simulink model "One_Pedal"  (R2024a)
settings: Solver=VariableStepAuto  StartTime=0.0  StopTime=10.0  RelTol=1e-3
undefined symbols (not defined in the file): Ion, Lithium
libraries: simulink x2, spsBatteryLib x1, spsControlledCurrentSourceLib x1, spsVoltageMeasurementLib x1, sps_lib x1
settings Model: Creator=ezeki  LastModifiedBy=ezeki

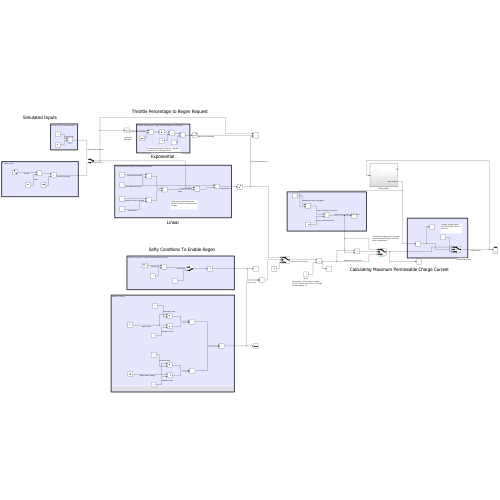
[thumbnail: Simulink's stored preview of the top-level diagram]
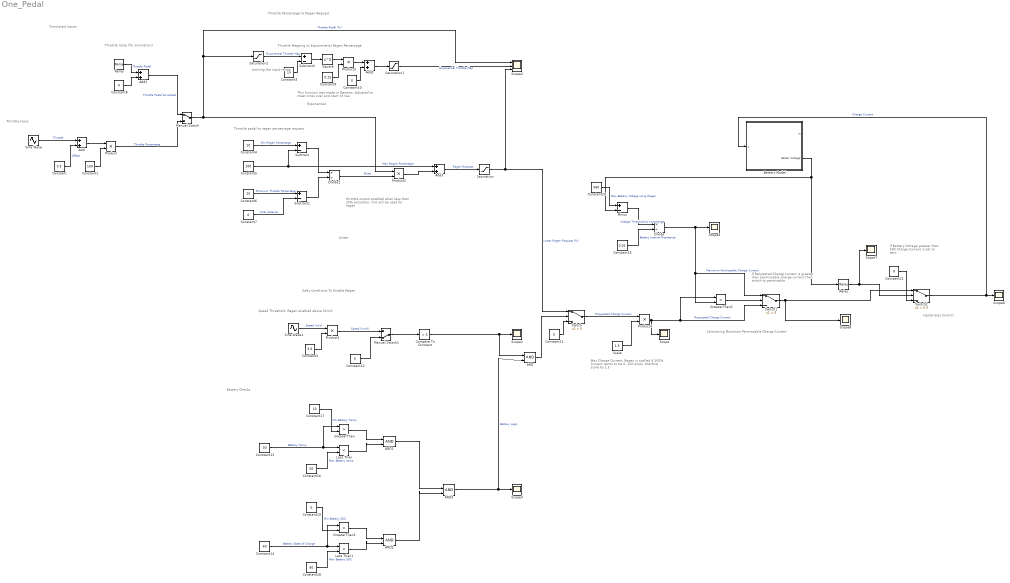
== system One_Pedal ==
  note: Linear
  note: Calculating Maximum Permissable Charge Current
  note: Throttle Percentage to Regen Request
  note: Simulated Inputs
  note: Safty Condtions To Enable Regen
  note: Max Charge Current, Regen is scalled 0-100%. Current wants to be 0 -150 amps, therfore scale by 1.5
  note: Battery Checks
  note: This function was made in Desmos. Adjusted to meet cross over and start of rise
  note: Limiting the input range
  note: Throttle Mapping to Exponenetial Regen Percentage
  note: Throttle ramp (for simulation)
  note: Throttle pedal to regen percentage request
  note: throttle output enabled when less then 20% actuation, this will be used for regen
  note: Speed Threshold, Regen enabled above 5km/h
  note: Throttle Input
  note: Hysterisies Control
  note: If Requested Charge current is greater then permissable charge current then switch to permisable
  note: If Battery Voltage greater then 590 Charge Current is set to zero
  note: Exponential
  AND{,1..3} (4 alike) : Logic  IconShape=distinctive  AllPortsSameDT=off  OutDataTypeStr=boolean
  Add{,1..3} (4 alike) : Sum
  Battery Model : Subsystem
  Compare To Constant : simulink/Logic and Bit Operations/Compare To Constant  relop=>  const=5  OutDataTypeStr=boolean
  Constant : Constant  Value=0.5
  Constant1 : Constant  Value=100
  Constant{7..8,10..11,21} (5 alike) : Constant  Value=0
  Constant12 : Constant  Value=6
  Constant13 : Constant  Value=30
  Constant14 : Constant  Value=60
  Constant15 : Constant  Value=0.01
  Constant16 : Constant  Value=50
  Constant17 : Constant  Value=10
  Constant18 : Constant  Value=90
  Constant19 : Constant  Value=5
  Constant2 : Constant  Value=3.6
  Constant20 : Constant  Value=580
  Constant3 : Constant  Value=20
  Constant4 : Constant  Value=10
  Constant5 : Constant  Value=100
  Constant6 : Constant  Value=20
  Constant9 : Constant  Value=0.25
  Divide : Product  Inputs=*/
  Divide1 : Product  Inputs=*/
  GreaterThan : RelationalOperator  Operator=>  OutDataTypeStr=boolean  RndMeth=Simplest  InputSameDT=off
  GreaterThan1 : RelationalOperator  Operator=>  OutDataTypeStr=boolean  RndMeth=Simplest  InputSameDT=off
  GreaterThan2 : RelationalOperator  Operator=>  OutDataTypeStr=boolean  RndMeth=Simplest  InputSameDT=off
  Less Than : RelationalOperator  Operator=<  OutDataTypeStr=boolean  RndMeth=Simplest  InputSameDT=off
  Less Than1 : RelationalOperator  Operator=<  OutDataTypeStr=boolean  RndMeth=Simplest  InputSameDT=off
  Manual Switch : ManualSwitch
  Manual Switch1 : ManualSwitch  CurrentSetting=0
  Minus : Sum  Inputs=+-
  Product{,1..4} (5 alike) : Product
  Ramp : simulink/Sources/Ramp  slope=-10  start=0  InitialOutput=100
  Relay : Relay  OnSwitchValue=590  OffSwitchValue=585  OnOutputValue=0  OffOutputValue=1
  Saturation : Saturate  UpperLimit=100  LowerLimit=0
  Saturation1 : Saturate  UpperLimit=100  LowerLimit=0
  Saturation2 : Saturate  UpperLimit=20  LowerLimit=0
  Scale : Constant  Value=1.5
  Scope{,1,3,6..9} (7 alike) : Scope
  Scope2 : Scope  NumInputPorts=3
  Sine Wave : Sin  Amplitude=0.5  SampleTime=0
  Sine Wave1 : Sin  SampleTime=0
  Square : Math  Operator=square
  Subtract : Sum  Inputs=+-
  Subtract1 : Sum  Inputs=+-
  Subtract2 : Sum  Inputs=+-
  Switch : Switch  Criteria=u2 > Threshold  SaturateOnIntegerOverflow=off  InputSameDT=off
  Switch1 : Switch  Criteria=u2 > Threshold  SaturateOnIntegerOverflow=off  InputSameDT=off
  Switch2 : Switch  Criteria=u2 > Threshold  Threshold=0.5  SaturateOnIntegerOverflow=off  InputSameDT=off
  wires:
  Sine Wave/1 -> Add/1  "Throttle"
  Constant/1 -> Add/2  "Offset"
  Constant1/1 -> Product/2
  Add/1 -> Product/1
  Product/1 -> Manual Switch/2  "Throttle Percentage"
  Sine Wave1/1 -> Product1/1  "Speed (m/s)"
  Constant2/1 -> Product1/2
  Product1/1 -> Manual Switch1/1  "Speed (km/h)"
  Compare To Constant/1 -> AND/1, Scope1/1
  Constant7/1 -> Subtract1/2  "Intial distance"
  Constant4/1 -> Subtract/1  "Min Regen Percentage"
  Constant6/1 -> Subtract1/1  "Minimum Throttle Percentage"
  Subtract/1 -> Divide1/1
  Constant5/1 -> Subtract/2, Add3/1  "Max Regen Percentage"
  Divide1/1 -> Product2/2  "Slope"
  Product2/1 -> Add3/2
  Subtract1/1 -> Divide1/2
  Add3/1 -> Saturation/1  "Regen Request"
  Manual Switch/1 -> Scope2/1, Saturation2/1, Product2/1  "Throttle Pedal (%)"
  Ramp/1 -> Add1/1  "Throttle Pedal"
  Constant8/1 -> Add1/2
  Add1/1 -> Manual Switch/1  "Throttle Pedal Simulated"
  Saturation/1 -> Switch/1, Scope2/3  "Linear Regen Request (%)"
  Subtract2/1 -> Square/1
  Constant3/1 -> Subtract2/2
  Add2/1 -> Saturation1/1
  Square/1 -> Product3/1
  Constant9/1 -> Product3/2
  Product3/1 -> Add2/1
  Constant10/1 -> Add2/2
  Saturation2/1 -> Subtract2/1  "Exponential Throttle Map"
  Constant11/1 -> Switch/3
  Manual Switch1/1 -> Compare To Constant/1
  Constant12/1 -> Manual Switch1/2
  AND/1 -> Switch/2
  Constant13/1 -> GreaterThan/1, Less Than/1  "Battery Temp"
  Constant14/1 -> GreaterThan1/1, Less Than1/1  "Battery State of Charge"
  AND3/1 -> Scope3/1, AND/2  "Battery Logic"
  Constant16/1 -> Less Than/2  "Max Battery temp"
  Constant17/1 -> GreaterThan/2  "Min Battery Temp"
  GreaterThan/1 -> AND1/1
  Less Than/1 -> AND1/2
  Constant19/1 -> GreaterThan1/2  "Min Battery SOC"
  GreaterThan1/1 -> AND2/1
  Constant18/1 -> Less Than1/2  "Max Battery SOC"
  Less Than1/1 -> AND2/2
  AND1/1 -> AND3/1
  AND2/1 -> AND3/2
  Switch2/1 -> Battery Model/1(s), Scope6/1  "Charge Current"
  Product4/1 -> Switch1/3, GreaterThan2/1, Scope/1  "Requested Charge Current"
  Divide/1 -> GreaterThan2/2, Switch1/1, Scope9/1  "Maximum Permissable Charge Current"
  Constant15/1 -> Divide/2  "Battery Internal Resistance"
  Battery Model/2(Batter Voltage) -> Minus/2, Relay/1
  Relay/1 -> Switch2/2, Scope7/1
  Constant21/1 -> Switch2/3
  Switch1/1 -> Switch2/1, Scope8/1
  Minus/1 -> Divide/1  "Voltage Threshold to overcharge"
  GreaterThan2/1 -> Switch1/2
  Constant20/1 -> Minus/1  "Max Battery Voltage using Regen"
  Switch/1 -> Product4/1  "Requested Charge Current"
  Scale/1 -> Product4/2
  Saturation1/1 -> Scope2/2  "Exponential Throttle Map"

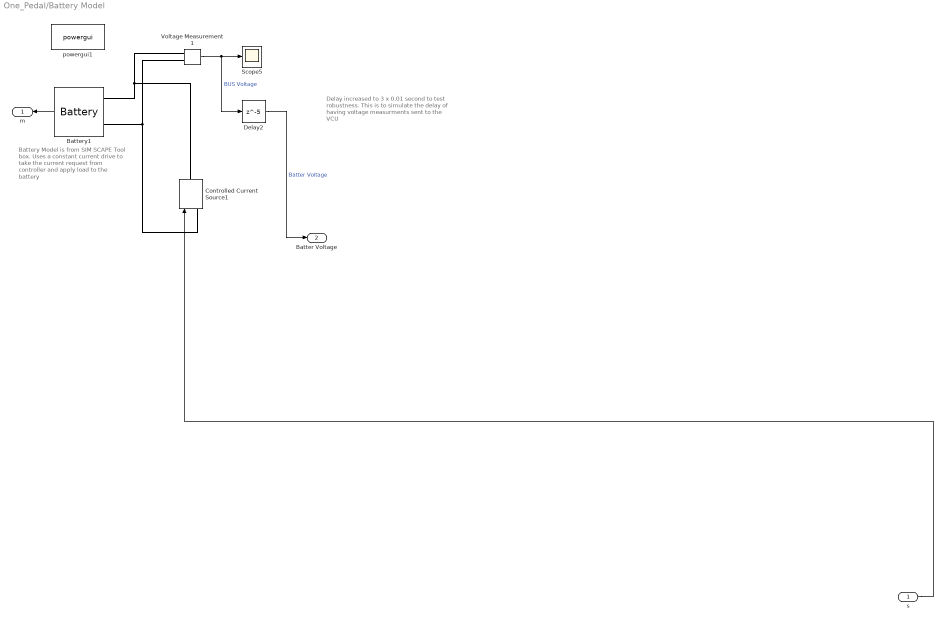
== system One_Pedal/Battery Model ==
  note: Delay increased to 3 x 0.01 second to test robustness. This is to simulate the delay of having voltage measurments sent to the VCU
  note: Battery Model is from SIM SCAPE Tool box. Uses a constant current drive to take the current request from controller and apply load to the battery
  s : Inport
  Battery1 : spsBatteryLib/Battery  BatType=Lithium-Ion  ShowTempParam=off  ThermalPreset=no  ShowAgeParam=off  NomV=532.8  NomQ=1152  SOC=85  Batt_Tr=5  PresetModel=on  MaxQ=1152  MinV=399.6  FullV=620.1723  Dis_rate=500.8696  R=0.004625  Normal_OP=1041.8087  expZone="[575.6296      56.59826]"  current=[6.5 13 32.5]  Units=Time  Tci=20  NomT=20  T2=-30  MaxQ2=4.8  FullV2=7.1  Normal_OP2=5.655  expZone2="[6.58           1]"  Rca=0.6  ti=2000  Dp=0  Neq0=0  Tsim=1e6  Ta1=25  Qeol=5.4*0.9  Reol=0.013333*1.2  Char_age=[2.3478, 3]  Dis_age=[2.3478, 10]  N1=1500  N2=10500  N3=1000  N4=1400  Ta2=45  N5=950
  Controlled Current Source1 : spsControlledCurrentSourceLib/Controlled Current Source  Initialize=on  Source_Type=AC  Amplitude=0  Phase=0  Frequency=0  Measurements=None
  Delay2 : Delay  DelayLength=5  InitialCondition=580
  Scope5 : Scope
  Voltage Measurement1 : spsVoltageMeasurementLib/Voltage Measurement  PhasorSimulation=off  OutputType=Complex  PSBequivalent=0
  powergui1 : sps_lib/powergui  Priority=1  SimulationMode=Discrete  SampleTime=0.01  frequency=60  Iterations=50  frequencyindice=0  Pbase=100e6  ErrMax=1e-4  UnitsV=kV  UnitsW=MW  buscounter=0  FunctionMessages=off  echomessages=off  EnableUseOfTLC=off  CurrentSourceSwitches=off  DisableSnubberDevices=off  DisableRonSwitches=off  DisableVfSwitches=off  DisplayEquations=off  AutomaticDiscreteSolvers=off  SolverType=Tustin/Backward Euler (TBE)  Interpol=off  ExternalGateDelay=off  methode=off  Ts=100  x0status=blocks  SPID=on  SwTol=0  HookPort=off  NonlinearTolerance=1e-4  nMaxIteration=100  ContinueOnMaxIteration=off  RestoreLinks=warning  ResistiveCurrentMeasurement=off  Frange=[0:2:500]  Ylog=off  Xlog=on  ShowGrid=off  save=off  variable=ZData  structure=0  ZoomFFT=off  StartTime=0.0  cycles=1  DisplayStyle=1  fundamental=60  FreqAxis=off  MaxFrequency=1000  frequencyindicesteady=1  RmsSteady=1  display=off
  m : Outport
  Batter Voltage : Outport  Port=2
  wires:
  Voltage Measurement1/1 -> Delay2/1, Scope5/1  "BUS Voltage"
  s/1 -> Controlled Current Source1/1
  Delay2/1 -> Batter Voltage/1  "Batter Voltage"
  Battery1/1 -> m/1
  connections:
  Voltage Measurement1/LConn1 -- Controlled Current Source1/RConn1 -- Battery1/LConn1
  Battery1/LConn2 -- Voltage Measurement1/LConn2 -- Controlled Current Source1/LConn1
